simulink model "FixedWingSim_SimulinkDiagram"  (R2024a)
settings: Solver=ode5  StartTime=0.0  StopTime=100.0  FixedStep=0.01  RelTol=1e-3  EnableMultiTasking=on
values from neighbouring files (symbols this model uses):
  a = da0    [FixedWingSim_Main.m]
  alpha0 = 3.6102915*d2r    (= 0.0630114736318)    [FixedWingSim_Parameters.m]
  b = 30.0    (= 30)    [FixedWingSim_Parameters.m]
  beta0 = 0.0    (= 0)    [FixedWingSim_Parameters.m]
  cbar = 11.32    [FixedWingSim_Parameters.m]
  CDa = 0.00550063/d2r    (= 0.315162883663)    [FixedWingSim_Parameters.m]
  CDadot = 0.0    (= 0)    [FixedWingSim_Parameters.m]
  CDde = -0.000587647/d2r    (= -0.0336696929435)    [FixedWingSim_Parameters.m]
  CDdf = 0.00136385/d2r    (= 0.0781428488889)    [FixedWingSim_Parameters.m]
  CDo = 0.01192128    [FixedWingSim_Parameters.m]
  CDq = 0.00315057/d2r    (= 0.180514364061)    [FixedWingSim_Parameters.m]
  CLa = 0.0794655/d2r    (= 4.5530377669)    [FixedWingSim_Parameters.m]
  CLadot = 0.0    (= 0)    [FixedWingSim_Parameters.m]
  Clb = -0.00173748/d2r    (= -0.0995502709884)    [FixedWingSim_Parameters.m]
  Clda = -0.00213984/d2r    (= -0.122603800833)    [FixedWingSim_Parameters.m]
  CLde = 0.0121988/d2r    (= 0.698939755124)    [FixedWingSim_Parameters.m]
  CLdf = 0.0144389/d2r    (= 0.827288030811)    [FixedWingSim_Parameters.m]
  Cldr = 0.000479021/d2r    (= 0.0274458815981)    [FixedWingSim_Parameters.m]
  CLo = 0.004608463    [FixedWingSim_Parameters.m]
  Clo = 0.0    (= 0)    [FixedWingSim_Parameters.m]
  Clp = -0.00739342/d2r    (= -0.423611762168)    [FixedWingSim_Parameters.m]
  CLq = 0.0508476/d2r    (= 2.91335287837)    [FixedWingSim_Parameters.m]
  Clr = 0.0000699792/d2r    (= 0.0040095128137)    [FixedWingSim_Parameters.m]
  CMa = -0.0041873/d2r    (= -0.239914617555)    [FixedWingSim_Parameters.m]
  CMadot = -0.05/d2r    (= -2.86478897565)    [FixedWingSim_Parameters.m]
  CMde = -0.0115767/d2r    (= -0.663296050689)    [FixedWingSim_Parameters.m]
  CMdf = 0.000580220/d2r    (= 0.0332441571891)    [FixedWingSim_Parameters.m]
  CMo = -0.02092347    [FixedWingSim_Parameters.m]
  CMq = -0.060661/d2r    (= -3.47561928104)    [FixedWingSim_Parameters.m]
  CNb = 0.00320831/d2r    (= 0.18382262237)    [FixedWingSim_Parameters.m]
  CNda = -0.000206591/d2r    (= -0.0118367923854)    [FixedWingSim_Parameters.m]
  CNdr = -0.00144865/d2r    (= -0.0830015309916)    [FixedWingSim_Parameters.m]
  CNo = 0.0    (= 0)    [FixedWingSim_Parameters.m]
  CNp = -0.000432575/d2r    (= -0.0247847218229)    [FixedWingSim_Parameters.m]
  CNr = -0.00886783/d2r    (= -0.508089232439)    [FixedWingSim_Parameters.m]
  CYb = -0.0219309/d2r    (= -1.25654801092)    [FixedWingSim_Parameters.m]
  CYda = 0.00049355/d2r    (= 0.0282783319787)    [FixedWingSim_Parameters.m]
  CYdr = 0.00293048/d2r    (= 0.167904135947)    [FixedWingSim_Parameters.m]
  CYo = 0.0    (= 0)    [FixedWingSim_Parameters.m]
  CYp = 0.00133787/d2r    (= 0.0766543045372)    [FixedWingSim_Parameters.m]
  CYr = 0.0094053/d2r    (= 0.538883995054)    [FixedWingSim_Parameters.m]
  da0 = 0.0    (= 0)    [FixedWingSim_Parameters.m]
  de0 = -3.03804303*d2r    (= -0.0530238536908)    [FixedWingSim_Parameters.m]
  df0 = 1.5*d2r    (= 0.0261799387799)    [FixedWingSim_Parameters.m]
  dr0 = 0.0    (= 0)    [FixedWingSim_Parameters.m]
  e = de0    [FixedWingSim_Main.m]
  Ixx = 8890.63    [FixedWingSim_Parameters.m]
  Ixy = 0.0    (= 0)    [FixedWingSim_Parameters.m]
  Ixz = 181.119    [FixedWingSim_Parameters.m]
  Iyy = 71973.5    [FixedWingSim_Parameters.m]
  Iyz = 0.0    (= 0)    [FixedWingSim_Parameters.m]
  Izz = 77141.1    [FixedWingSim_Parameters.m]
  K = inv([ Ixx, -Ixy, -Ixz ... (first row only)    [FixedWingSim_Main.m]
  mass = 762.8447    [FixedWingSim_Parameters.m]
  p0 = 0.0    (= 0)    [FixedWingSim_Parameters.m]
  phi0 = 0.0    (= 0)    [FixedWingSim_Parameters.m]
  psi0 = 0.0    (= 0)    [FixedWingSim_Parameters.m]
  q0 = 0.0    (= 0)    [FixedWingSim_Parameters.m]
  r = dr0 - (2.0 * d2r)    [FixedWingSim_Main.m]
  r0 = 0.0    (= 0)    [FixedWingSim_Parameters.m]
  r2d = 180/pi    (= 57.2957795131)    [FixedWingSim_Parameters.m]
  S = 300.0    (= 300)    [FixedWingSim_Parameters.m]
  theta0 = alpha0    (= 0.0630114736318)    [FixedWingSim_Parameters.m]
  thrust = 3146.482666    [FixedWingSim_Parameters.m]
  Vt0 = 626.81863    [FixedWingSim_Parameters.m]
settings Model: Creator=Bryan Lukehart-Yun  LastModifiedBy=bryan
settings SolverCC: AlgebraicLoopSolver=TrustRegion
settings DebuggingCC: UnconnectedInputMsg=warning  UnconnectedOutputMsg=warning  UnconnectedLineMsg=warning
settings ModelReferenceCC: EnableRefExpFcnMdlSchedulingChecks=on
settings RTWCC: GPUComputeCapability=3.5

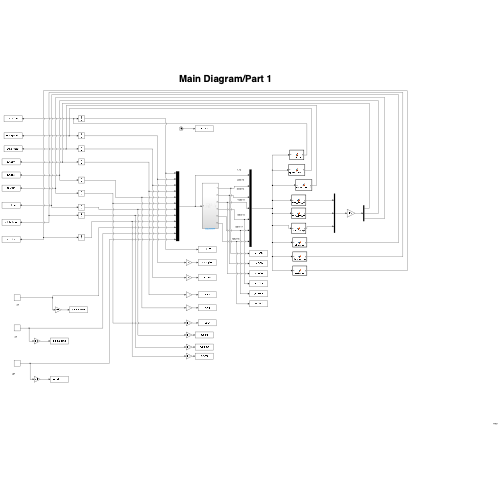
[thumbnail: Simulink's stored preview of the top-level diagram]
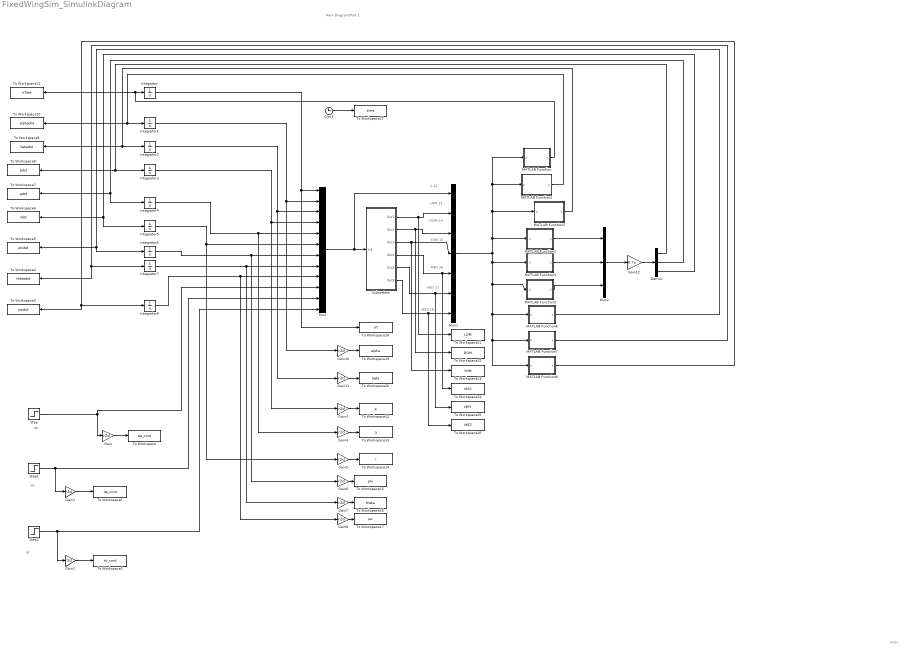
== system FixedWingSim_SimulinkDiagram ==
  note: de
  note: da
  note: dr
  note: MEZ 18
  note: MEY 17
  note: MEX 16
  note: YOM 15
  note: DOM 14
  note: LOM 13
  note: 1-12
  note: main
  note: Main Diagram/Part 1
  Clock : Clock
  Demux : Demux  Outputs=3
  Gain{,1..8,10..11} (11 alike) : Gain  Gain=r2d
  Gain12 : Gain  Gain=K  Multiplication=Matrix(K*u)
  Integrator : Integrator  InitialCondition=Vt0
  Integrator1 : Integrator  InitialCondition=alpha0
  Integrator2 : Integrator  InitialCondition=beta0
  Integrator3 : Integrator  InitialCondition=p0
  Integrator4 : Integrator  InitialCondition=q0
  Integrator5 : Integrator  InitialCondition=r0
  Integrator6 : Integrator  InitialCondition=phi0
  Integrator7 : Integrator  InitialCondition=theta0
  Integrator8 : Integrator  InitialCondition=psi0
  MATLAB Function : MATLAB Function  TreatAsAtomicUnit=on
  MATLAB Function1 : MATLAB Function  TreatAsAtomicUnit=on
  MATLAB Function2 : MATLAB Function  TreatAsAtomicUnit=on
  MATLAB Function3 : MATLAB Function  TreatAsAtomicUnit=on
  MATLAB Function4 : MATLAB Function  TreatAsAtomicUnit=on
  MATLAB Function5 : MATLAB Function  TreatAsAtomicUnit=on
  MATLAB Function6 : MATLAB Function  TreatAsAtomicUnit=on
  MATLAB Function7 : MATLAB Function  TreatAsAtomicUnit=on
  MATLAB Function8 : MATLAB Function  TreatAsAtomicUnit=on
  Mux : Mux  Inputs=12
  Mux1 : Mux  Inputs=7
  Mux2 : Mux  Inputs=3
  Step : Step  Before=de0  After=e  SampleTime=0
  Step1 : Step  Before=da0  After=a  SampleTime=0
  Step2 : Step  Before=dr0  After=r  SampleTime=0
  Subsystem : Subsystem  Description=Hi
  To Workspace : ToWorkspace  VariableName=de_cmd  SampleTime=-1
  To Workspace1 : ToWorkspace  VariableName=da_cmd  SampleTime=-1
  To Workspace10 : ToWorkspace  VariableName=alphadot  SampleTime=-1
  To Workspace11 : ToWorkspace  VariableName=VTdot  SampleTime=-1
  To Workspace12 : ToWorkspace  VariableName=p  SampleTime=-1
  To Workspace13 : ToWorkspace  VariableName=q  SampleTime=-1
  To Workspace14 : ToWorkspace  VariableName=r  SampleTime=-1
  To Workspace15 : ToWorkspace  VariableName=phi  SampleTime=-1
  To Workspace16 : ToWorkspace  VariableName=theta  SampleTime=-1
  To Workspace17 : ToWorkspace  VariableName=psi  SampleTime=-1
  To Workspace18 : ToWorkspace  VariableName=VT  SampleTime=-1
  To Workspace19 : ToWorkspace  VariableName=alpha  SampleTime=-1
  To Workspace2 : ToWorkspace  VariableName=dr_cmd  SampleTime=-1
  To Workspace20 : ToWorkspace  VariableName=beta  SampleTime=-1
  To Workspace21 : ToWorkspace  VariableName=LOM  SampleTime=-1
  To Workspace22 : ToWorkspace  VariableName=DOM  SampleTime=-1
  To Workspace23 : ToWorkspace  VariableName=YOM  SampleTime=-1
  To Workspace24 : ToWorkspace  VariableName=MEX  SampleTime=-1
  To Workspace25 : ToWorkspace  VariableName=MEY  SampleTime=-1
  To Workspace26 : ToWorkspace  VariableName=MEZ  SampleTime=-1
  To Workspace27 : ToWorkspace  VariableName=time  SampleTime=-1
  To Workspace3 : ToWorkspace  VariableName=psidot  SampleTime=-1
  To Workspace4 : ToWorkspace  VariableName=thetadot  SampleTime=-1
  To Workspace5 : ToWorkspace  VariableName=phidot  SampleTime=-1
  To Workspace6 : ToWorkspace  VariableName=rdot  SampleTime=-1
  To Workspace7 : ToWorkspace  VariableName=qdot  SampleTime=-1
  To Workspace8 : ToWorkspace  VariableName=pdot  SampleTime=-1
  To Workspace9 : ToWorkspace  VariableName=betadot  SampleTime=-1
  wires:
  Gain1/1 -> To Workspace1/1
  Gain/1 -> To Workspace/1
  Gain2/1 -> To Workspace2/1
  Gain4/1 -> To Workspace13/1
  Gain3/1 -> To Workspace12/1
  Gain5/1 -> To Workspace14/1
  Gain8/1 -> To Workspace17/1
  Gain7/1 -> To Workspace16/1
  Gain6/1 -> To Workspace15/1
  Gain11/1 -> To Workspace20/1
  Gain10/1 -> To Workspace19/1
  Mux/1 -> Mux1/1, Subsystem/1(In1)
  Mux1/1 -> MATLAB Function8/1(u), MATLAB Function7/1(u), MATLAB Function6/1(u), MATLAB Function5/1(u), MATLAB Function4/1(u), MATLAB Function1/1(u), MATLAB Function/1(u), MATLAB Function2/1(u), MATLAB Function3/1(u)
  Subsystem/1(Out1) -> To Workspace21/1, Mux1/2
  Subsystem/2(Out2) -> To Workspace22/1, Mux1/3
  Subsystem/3(Out3) -> To Workspace23/1, Mux1/4
  Subsystem/4(Out4) -> To Workspace24/1, Mux1/5
  Subsystem/5(Out5) -> To Workspace25/1, Mux1/6
  Subsystem/6(Out6) -> To Workspace26/1, Mux1/7
  Integrator/1 -> To Workspace18/1, Mux/1
  MATLAB Function/1(y) -> To Workspace11/1, Integrator/1
  MATLAB Function1/1(y) -> To Workspace10/1, Integrator1/1
  Integrator1/1 -> Gain10/1, Mux/2
  MATLAB Function2/1(y) -> To Workspace9/1, Integrator2/1
  Integrator2/1 -> Mux/3, Gain11/1
  Integrator3/1 -> Gain3/1, Mux/4
  MATLAB Function4/1(y) -> Mux2/2
  Mux2/1 -> Gain12/1
  MATLAB Function3/1(y) -> Mux2/1
  MATLAB Function5/1(y) -> Mux2/3
  Gain12/1 -> Demux/1
  Demux/1 -> Integrator3/1, To Workspace8/1
  Demux/2 -> To Workspace7/1, Integrator4/1
  Integrator4/1 -> Gain4/1, Mux/5
  Demux/3 -> To Workspace6/1, Integrator5/1
  Integrator5/1 -> Mux/6, Gain5/1
  Step/1 -> Mux/10, Gain/1
  Step1/1 -> Gain1/1, Mux/11
  Step2/1 -> Gain2/1, Mux/12
  Integrator6/1 -> Gain6/1, Mux/7
  MATLAB Function6/1(y) -> To Workspace5/1, Integrator6/1
  Integrator7/1 -> Gain7/1, Mux/8
  Integrator8/1 -> Gain8/1, Mux/9
  MATLAB Function7/1(y) -> To Workspace4/1, Integrator7/1
  MATLAB Function8/1(y) -> To Workspace3/1, Integrator8/1
  Clock/1 -> To Workspace27/1

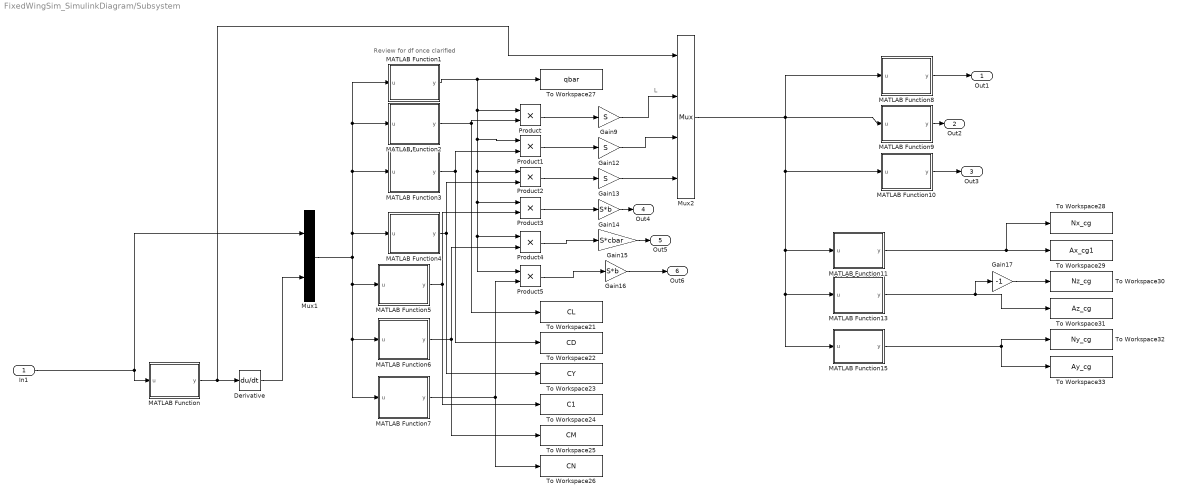
== system FixedWingSim_SimulinkDiagram/Subsystem ==
  note: Review for df once clarified
  note: L
  In1 : Inport
  Derivative : Derivative
  Gain12 : Gain  Gain=S
  Gain13 : Gain  Gain=S
  Gain14 : Gain  Gain=S*b
  Gain15 : Gain  Gain=S*cbar
  Gain16 : Gain  Gain=S*b
  Gain17 : Gain  Gain=-1
  Gain9 : Gain  Gain=S
  MATLAB Function : MATLAB Function  TreatAsAtomicUnit=on
  MATLAB Function1 : MATLAB Function  TreatAsAtomicUnit=on
  MATLAB Function10 : MATLAB Function  TreatAsAtomicUnit=on
  MATLAB Function11 : MATLAB Function  TreatAsAtomicUnit=on
  MATLAB Function13 : MATLAB Function  TreatAsAtomicUnit=on
  MATLAB Function15 : MATLAB Function  TreatAsAtomicUnit=on
  MATLAB Function2 : MATLAB Function  TreatAsAtomicUnit=on
  MATLAB Function3 : MATLAB Function  TreatAsAtomicUnit=on
  MATLAB Function4 : MATLAB Function  TreatAsAtomicUnit=on
  MATLAB Function5 : MATLAB Function  TreatAsAtomicUnit=on
  MATLAB Function6 : MATLAB Function  TreatAsAtomicUnit=on
  MATLAB Function7 : MATLAB Function  TreatAsAtomicUnit=on
  MATLAB Function8 : MATLAB Function  TreatAsAtomicUnit=on
  MATLAB Function9 : MATLAB Function  TreatAsAtomicUnit=on
  Mux1 : Mux  Inputs=2
  Mux2 : Mux
  Product{,1..5} (6 alike) : Product
  To Workspace21 : ToWorkspace  VariableName=CL  SampleTime=-1
  To Workspace22 : ToWorkspace  VariableName=CD  SampleTime=-1
  To Workspace23 : ToWorkspace  VariableName=CY  SampleTime=-1
  To Workspace24 : ToWorkspace  VariableName=C1  SampleTime=-1
  To Workspace25 : ToWorkspace  VariableName=CM  SampleTime=-1
  To Workspace26 : ToWorkspace  VariableName=CN  SampleTime=-1
  To Workspace27 : ToWorkspace  VariableName=qbar  SampleTime=-1
  To Workspace28 : ToWorkspace  VariableName=Nx_cg  SampleTime=-1
  To Workspace29 : ToWorkspace  VariableName=Ax_cg1  SampleTime=-1
  To Workspace30 : ToWorkspace  VariableName=Nz_cg  SampleTime=-1
  To Workspace31 : ToWorkspace  VariableName=Az_cg  SampleTime=-1
  To Workspace32 : ToWorkspace  VariableName=Ny_cg  SampleTime=-1
  To Workspace33 : ToWorkspace  VariableName=Ay_cg  SampleTime=-1
  Out1 : Outport
  Out2 : Outport  Port=2
  Out3 : Outport  Port=3
  Out4 : Outport  Port=4
  Out5 : Outport  Port=5
  Out6 : Outport  Port=6
  wires:
  Product/1 -> Gain9/1
  MATLAB Function4/1(y) -> To Workspace23/1, Product2/2
  MATLAB Function1/1(y) -> Product/1, Product1/1, Product2/1, Product3/1, Product4/1, Product5/1, To Workspace27/1
  Gain17/1 -> To Workspace30/1
  Mux1/1 -> MATLAB Function7/1(u), MATLAB Function6/1(u), MATLAB Function5/1(u), MATLAB Function4/1(u), MATLAB Function1/1(u), MATLAB Function2/1(u), MATLAB Function3/1(u)
  MATLAB Function13/1(y) -> Gain17/1, To Workspace31/1
  Gain9/1 -> Mux2/2
  MATLAB Function7/1(y) -> Product5/2, To Workspace26/1
  MATLAB Function11/1(y) -> To Workspace28/1, To Workspace29/1
  MATLAB Function5/1(y) -> To Workspace24/1, Product3/2
  MATLAB Function6/1(y) -> To Workspace25/1, Product4/2
  Mux2/1 -> MATLAB Function13/1(u), MATLAB Function15/1(u), MATLAB Function11/1(u), MATLAB Function10/1(u), MATLAB Function8/1(u), MATLAB Function9/1(u)
  MATLAB Function3/1(y) -> Product1/2, To Workspace22/1
  Product5/1 -> Gain16/1
  MATLAB Function8/1(y) -> Out1/1
  Product3/1 -> Gain14/1
  MATLAB Function2/1(y) -> Product/2, To Workspace21/1
  Product1/1 -> Gain12/1
  MATLAB Function10/1(y) -> Out3/1
  In1/1 -> MATLAB Function/1(u), Mux1/1
  MATLAB Function15/1(y) -> To Workspace32/1, To Workspace33/1
  Gain12/1 -> Mux2/3
  MATLAB Function9/1(y) -> Out2/1
  Gain13/1 -> Mux2/4
  Product2/1 -> Gain13/1
  Product4/1 -> Gain15/1
  Gain15/1 -> Out5/1
  Gain16/1 -> Out6/1
  Gain14/1 -> Out4/1
  Derivative/1 -> Mux1/2
  MATLAB Function/1(y) -> Mux2/1, Derivative/1

== matlab function FixedWingSim_SimulinkDiagram/Subsystem/MATLAB Function7 ==
  data: u input size=13; y output; CNo parameter; CNb parameter; b parameter; CNp parameter; CNr parameter; CNda parameter; CNdr parameter
function y = Cn_fcn(u,CNo, CNb, b, CNp, CNr, CNda, CNdr)

y =CNo+(CNb*u(3))+(b/(2*u(1)) )*(CNp*u(4)+CNr*u(6))+CNda*u(11)+CNdr*u(12);

== matlab function FixedWingSim_SimulinkDiagram/Subsystem/MATLAB Function10 ==
  data: u input size=4; y output; mass parameter
function y = YOM_fcn(u, mass)

y = u(4)/mass;

== matlab function FixedWingSim_SimulinkDiagram/Subsystem/MATLAB Function8 ==
  data: u input; y output; thrust parameter; mass parameter
function y = LOM_fcn(u,thrust,mass)
y=1;
y = (u(2)+thrust*sin(u(1)) )/mass;

== matlab function FixedWingSim_SimulinkDiagram/Subsystem/MATLAB Function9 ==
  data: u input; y output; thrust parameter; mass parameter
function y = DOM_fcn(u,thrust, mass)
y=1; 
y = (u(3)-thrust*cos(u(1)))/mass;

== matlab function FixedWingSim_SimulinkDiagram/Subsystem/MATLAB Function11 ==
  data: u input; y output
function y = X_fcn(u)

y = -u(3)*cos(u(1))+u(2)*sin(u(1));

== matlab function FixedWingSim_SimulinkDiagram/Subsystem/MATLAB Function13 ==
  data: u input; y output
function y = Z_fcn(u)

y =-u(3)*sin(u(1))-u(2)*cos(u(1));

== matlab function FixedWingSim_SimulinkDiagram/Subsystem/MATLAB Function15 ==
  data: u input; y output
function y = Y_fcn(u)

y = u(4);

== matlab function FixedWingSim_SimulinkDiagram/MATLAB Function ==
  data: u input size=18; y output; g parameter
function y = Vdot_fcn(u,g)
y=1;
y = u(15)*sin(u(3))-u(14)*cos(u(3))+g*((cos(u(8))*cos(u(7))*sin(u(2))-sin(u(8))*cos(u(2)))*cos(u(3))+cos(u(8))*sin(u(7))*sin(u(3)));

== matlab function FixedWingSim_SimulinkDiagram/Subsystem/MATLAB Function1 ==
  data: u input; y output; rho parameter
function y = qbar_fcn(u, rho)
y=1; 
y= 0.5*rho*u(1)^2;

== matlab function FixedWingSim_SimulinkDiagram/MATLAB Function1 ==
  data: u input; y output; g parameter
function y = alphadot_ans_fcn(u,g)
y=1; 
y = u(5)-tan(u(3))*( u(4)*cos(u(2))+u(6)*sin(u(4)))-(u(13)/(u(1)*cos(u(3))))+(g/(u(1)*cos(u(3))) )*(cos(u(8))*cos(u(7))*cos(u(2))+sin(u(8))*sin(u(2)));

== matlab function FixedWingSim_SimulinkDiagram/MATLAB Function2 ==
  data: u input; y output; g parameter
function y = betadot_ans_fcn(u,g)
y=1;
y=u(4)*sin(u(2))-u(6)*cos(u(2))+(1/u(1))*(u(15)*cos(u(3))+u(14)*sin(u(3)) )+(g/u(1))*(cos(u(8))*sin(u(7))*cos(u(3))+sin(u(8))*sin(u(3))*cos(u(2))-cos(u(8))*cos(u(7))*sin(u(3))*sin(u(2)));

== matlab function FixedWingSim_SimulinkDiagram/MATLAB Function3 ==
  data: u input; y output; Iyy parameter; Izz parameter; Iyz parameter; Ixy parameter; Ixz parameter
function y = RHS_pdot_fcn(u,Iyy, Izz, Iyz, Ixy, Ixz)
y=1;
y = (u(5)*u(6)*(Iyy-Izz) )+(u(5)^2-u(6)^2)*Iyz-(u(4)*u(6)*Ixy)+(u(4)*u(5)*Ixz)+u(16);

== matlab function FixedWingSim_SimulinkDiagram/MATLAB Function4 ==
  data: u input; y output; Izz parameter; Ixx parameter; Ixz parameter; Iyz parameter; Ixy parameter
function y = RHS_qdot_fcn(u,Izz, Ixx, Ixz, Iyz, Ixy)
y=1; 
y =u(4)*u(6)*(Izz-Ixx)+(u(6)^2-u(4)^2)*Ixz-u(4)*u(5)*Iyz+u(5)*u(6)*Ixy+u(17);

== matlab function FixedWingSim_SimulinkDiagram/MATLAB Function5 ==
  data: u input; y output; Ixx parameter; Iyy parameter; Ixy parameter; Ixz parameter; Iyz parameter
function y = RHS_rdot_fcn(u,Ixx, Iyy, Ixy, Ixz, Iyz)
y=1;
y =u(4)*u(5)*(Ixx-Iyy)+(u(4)^2-u(5)^2)*Ixy-u(5)*u(6)*Ixz+u(4)*u(6)*Iyz+u(18);

== matlab function FixedWingSim_SimulinkDiagram/MATLAB Function6 ==
  data: u input; y output
function y = phidot_fcn(u)
y=1;
y = u(4)+u(5)*sin(u(7))*tan(u(8))+u(6)*cos(u(7))*tan(u(8));

== matlab function FixedWingSim_SimulinkDiagram/MATLAB Function7 ==
  data: u input; y output
function y = theta_dot_fcn(u)
y=1; 
y = u(5)*cos(u(7))-u(6)*sin(u(7));

== matlab function FixedWingSim_SimulinkDiagram/MATLAB Function8 ==
  data: u input; y output
function y = psidot_fcn(u)
y=1; 
y = ( u(5)*sin(u(7))+u(6)*cos(u(7)) )*(1/cos(u(8)));

== matlab function FixedWingSim_SimulinkDiagram/Subsystem/MATLAB Function ==
  data: u input; y output
function y = alpha_fcn(u)
y=1; 
y = u(2);

== matlab function FixedWingSim_SimulinkDiagram/Subsystem/MATLAB Function2 ==
  data: u input; y output; CLo parameter; CLa parameter; cbar parameter; CLq parameter; CLadot parameter; CLde parameter; CLdf parameter; df0 parameter
function y = CL_fcn(u, CLo, CLa, cbar, CLq, CLadot, CLde,CLdf,df0)
y=1;
y = CLo+(CLa*u(2))+(cbar/(2*u(1)) )*(CLq*u(5)+CLadot*u(13))+CLde*u(10)+CLdf*df0;

== matlab function FixedWingSim_SimulinkDiagram/Subsystem/MATLAB Function3 ==
  data: u input; y output; CDo parameter; CDa parameter; cbar parameter; CDq parameter; CDadot parameter; CDde parameter; CDdf parameter; df0 parameter
function y = CD_fcn(u,CDo, CDa, cbar, CDq, CDadot, CDde,CDdf,df0)

y = CDo+CDa*u(2)+(cbar/(2*u(1)) )*(CDq*u(5)+CDadot*u(13))+CDde*u(10)+CDdf*df0;

== matlab function FixedWingSim_SimulinkDiagram/Subsystem/MATLAB Function4 ==
  data: u input; y output; CYo parameter; CYb parameter; CYp parameter; CYr parameter; CYda parameter; CYdr parameter; b parameter
function y = CY_fcn(u, CYo, CYb, CYp, CYr, CYda, CYdr, b)
y=1; 
y =CYo+CYb*u(3)+(b/(2*u(1)))*(CYp*u(4)+CYr*u(6))+CYda*u(11)+CYdr*u(12);

== matlab function FixedWingSim_SimulinkDiagram/Subsystem/MATLAB Function5 ==
  data: u input; y output; Clo parameter; Clb parameter; Clp parameter; Clr parameter; Clda parameter; Cldr parameter; b parameter
function y = Cl_fcn(u,Clo, Clb, Clp, Clr, Clda, Cldr,b)
y=1;
y = Clo+Clb*u(3)+(b/(2*u(1)))*(Clp*u(4)+Clr*u(6))+Clda*u(11)+Cldr*u(12);

== matlab function FixedWingSim_SimulinkDiagram/Subsystem/MATLAB Function6 ==
  data: u input; y output; CMa parameter; cbar parameter; CMq parameter; CMadot parameter; CMde parameter; CMdf parameter; CMo parameter; df0 parameter
function y = Cm_fcn(u,CMa, cbar, CMq, CMadot, CMde,CMdf, CMo,df0)
y=1;
y =CMo+CMa*u(2)+(cbar/(2*u(1)) )*(CMq*u(5)+CMadot*u(13))+CMde*u(10)+CMdf*df0;
